simulink model "model_controllers"  (R2019a)
settings: Solver=VariableStepAuto  StartTime=0.0  StopTime=1.2  FixedStep=1e-6  RelTol=1e-5
values from neighbouring files (symbols this model uses):
  Bm = 0.0022    [State_of_Art.m]    (also in results_plotter_one_run20.m)
  Jm = 0.0004    [State_of_Art.m]    (also in results_plotter_one_run20.m)
  k1 = OBL_HSO    [State_of_Art.m]    (also in results_plotter_one_run20.m = kEO)
  k2 = HSO    [State_of_Art.m]    (also in results_plotter_one_run20.m = kPSO)
  k3 = ASO    [State_of_Art.m]    (also in results_plotter_one_run20.m = kSanTLBO)
  k4 = SFS    [State_of_Art.m]    (also in results_plotter_one_run20.m = kDE)
  k5 = GWO    [State_of_Art.m]    (also in results_plotter_one_run20.m = kGA)
  k6 = OBL_HGSO    [results_plotter_one_run20.m]
  k7 = HGSO    [results_plotter_one_run20.m]
  Kb = 0.05    [State_of_Art.m]    (also in results_plotter_one_run20.m)
  Kt = 0.015    [State_of_Art.m]    (also in results_plotter_one_run20.m)
  La = 2.7    [State_of_Art.m]    (also in results_plotter_one_run20.m)
  Ra = 0.4    [State_of_Art.m]    (also in results_plotter_one_run20.m)
libraries: simulink x7, fuzblock x1
settings Model: Creator=Nelson Manuel  LastModifiedBy=Nelson Manuel

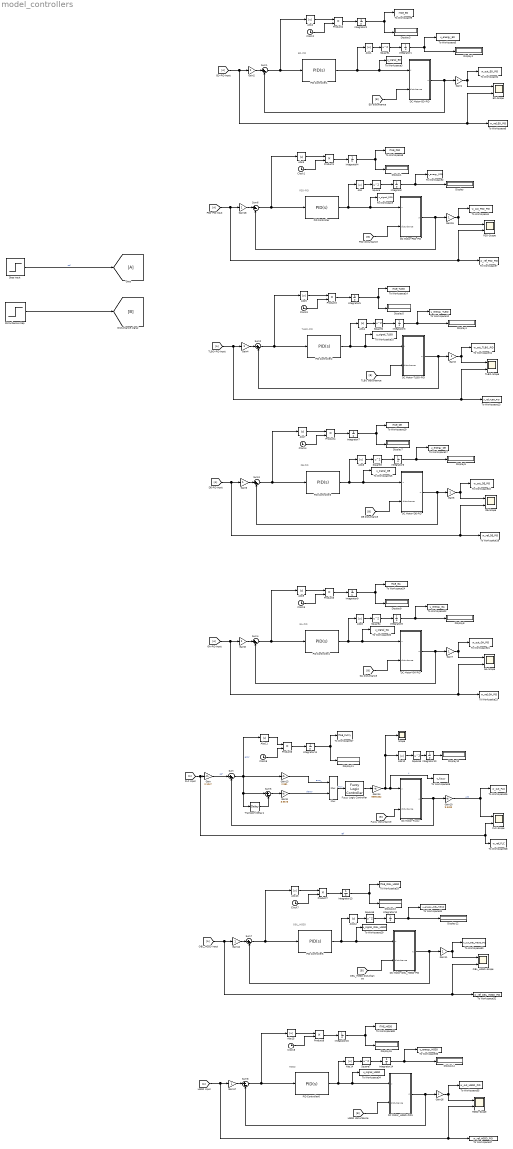
== system model_controllers ==
  note: EO-PID
  note: PSO-PID
  note: TLBO-PID
  note: DE-PID
  note: GA-PID
  note: OBL_HGSO
  note: HGSO
  Abs{,1..15} (16 alike) : Abs
  Clock{1..8} (8 alike) : Clock
  DC Motor-DE-PID : Subsystem
  DC Motor-EO-PID : Subsystem
  DC Motor-Fuzzy : Subsystem
  DC Motor-GA-PID : Subsystem
  DC Motor-OBL_HGSO-PID : Subsystem
  DC Motor-PSO-PID : Subsystem
  DC Motor-TLBO-PID : Subsystem
  DC Motor_HGSO-PID1 : Subsystem
  DE-Scope : Scope  NumInputPorts=2
  Display{,1..15} (16 alike) : Display
  Disturbance step : Step  Time=0  After=0  SampleTime=0
  EO-Scope : Scope  NumInputPorts=2
  FLC-Scope : Scope  NumInputPorts=2
  Fuzzy Logic Controller : fuzblock/Fuzzy Logic  Controller  FIS=FLC_Controller_updated  OutputSampleNumber=101  DataType=double  FuzzifiedInputs=off  RuleFiringStrengths=off  RuleOutputs=off  AggregatedOutputs=off  SimulateUsing=Interpreted execution  OutOfRangeInputValueMessage=none  NoRuleFiredMessage=none  EmptyOutputFuzzySetMessage=none
  GA-Scope : Scope  NumInputPorts=2
  Gain : Gain  Gain=0.1047
  Gain{1..8,11..12,15..18} (14 alike) : Gain
  Gain10 : Gain  Gain=9.5493
  Gain13 : Gain  Gain=2.981
  Gain14 : Gain  Gain=9999.852
  Gain9 : Gain  Gain=8.9578
  HGSO-Scope : Scope  NumInputPorts=2
  Integrator{,1..15} (16 alike) : Integrator
  Mux : Mux  Inputs=2
  OBL_HGSO-Scope : Scope  NumInputPorts=2
  PID Controller : simulink/Continuous/PID Controller  Controller=PID  Form=Parallel  TimeDomain=Continuous-time  SampleTime=-1  IntegratorMethod=Forward Euler  FilterMethod=Forward Euler  ControllerParametersSource=internal  P=k2(1)  I=k2(2)  D=k2(3)  UseFilter=on  N=1000  TunerSelectOption=Transfer Function Based (PID Tuner App)  InitialConditionSource=internal  InitialConditionForIntegrator=0  InitialConditionForFilter=0  DifferentiatorICPrevScaledInput=0  ExternalReset=none  TrackingMode=off  Kt=1  LimitOutput=off  UpperSaturationLimit=inf  LowerSaturationLimit=-inf  LinearizeAsGain=on  AntiWindupMode=none  Kb=1  POutMin=[]  POutMax=[]  IOutMin=[]  IOutMax=[]  DOutMin=[]  DOutMax=[]  NOutMin=[]  NOutMax=[]  SumOutMin=[]  SumOutMax=[]  SaturationOutMin=[]  SaturationOutMax=[]  PParamMin=[]  PParamMax=[]  IParamMin=[]  IParamMax=[]  DParamMin=[]  DParamMax=[]  NParamMin=[]  NParamMax=[]  KbParamMin=[]  KbParamMax=[]  KtParamMin=[]  KtParamMax=[]  KbOutMin=[]  KbOutMax=[]  KtOutMin=[]  KtOutMax=[]  IntegratorOutMin=[]  IntegratorOutMax=[]  FilterOutMin=[]  FilterOutMax=[]  SumI1OutMin=[]  SumI1OutMax=[]  SumI2OutMin=[]  SumI2OutMax=[]  SumI3OutMin=[]  SumI3OutMax=[]  SumI4OutMin=[]  SumI4OutMax=[]  SumDOutMin=[]  SumDOutMax=[]  DifferentiatorOutMin=[]  DifferentiatorOutMax=[]  FilterDiffOutCoefMin=[]  FilterDiffOutCoefMax=[]  ReciprocalOutMin=[]  ReciprocalOutMax=[]  SumDenOutMin=[]  SumDenOutMax=[]  SumNumOutMin=[]  SumNumOutMax=[]  DivideOutMin=[]  DivideOutMax=[]  IntegratorContinuousStateAttributes=''  IntegratorStateMustResolveToSignalObject=off  IntegratorRTWStateStorageClass=Auto  FilterContinuousStateAttributes=''  FilterStateMustResolveToSignalObject=off  FilterRTWStateStorageClass=Auto  ParallelPVariant=InternalParameters  IdealPVariant=Disabled  IVariant=InternalParameters  DVariant=InternalParameters  IntegratorVariant=Continuous  SatVariant=Disabled  AWVariant=Passthrough  PCopyVariant=Disabled  TRVariant=Disabled  FdbkBlocksVariant=Forward  IdealPFdbkVariant=Disabled  SatFdbkVariant=Disabled  DerivativeFilterVariant=ContFilter  NVariant=InternalParameters  NCopyVariant=Disabled  FilterICVariant=InternalICsFilter  IntegratorICVariant=InternalICs  ExternalResetVariant=Disabled  TRSumVariant=Passthrough  SumFdbkVariant=Disabled  SumVariant=Sum_PID
  PID Controller1 : simulink/Continuous/PID Controller  Controller=PID  Form=Parallel  TimeDomain=Continuous-time  SampleTime=-1  IntegratorMethod=Forward Euler  FilterMethod=Forward Euler  ControllerParametersSource=internal  P=k1(1)  I=k1(2)  D=k1(3)  UseFilter=on  N=1000  TunerSelectOption=Transfer Function Based (PID Tuner App)  InitialConditionSource=internal  InitialConditionForIntegrator=0  InitialConditionForFilter=0  DifferentiatorICPrevScaledInput=0  ExternalReset=none  TrackingMode=off  Kt=1  LimitOutput=off  UpperSaturationLimit=inf  LowerSaturationLimit=-inf  LinearizeAsGain=on  AntiWindupMode=none  Kb=1  POutMin=[]  POutMax=[]  IOutMin=[]  IOutMax=[]  DOutMin=[]  DOutMax=[]  NOutMin=[]  NOutMax=[]  SumOutMin=[]  SumOutMax=[]  SaturationOutMin=[]  SaturationOutMax=[]  PParamMin=[]  PParamMax=[]  IParamMin=[]  IParamMax=[]  DParamMin=[]  DParamMax=[]  NParamMin=[]  NParamMax=[]  KbParamMin=[]  KbParamMax=[]  KtParamMin=[]  KtParamMax=[]  KbOutMin=[]  KbOutMax=[]  KtOutMin=[]  KtOutMax=[]  IntegratorOutMin=[]  IntegratorOutMax=[]  FilterOutMin=[]  FilterOutMax=[]  SumI1OutMin=[]  SumI1OutMax=[]  SumI2OutMin=[]  SumI2OutMax=[]  SumI3OutMin=[]  SumI3OutMax=[]  SumI4OutMin=[]  SumI4OutMax=[]  SumDOutMin=[]  SumDOutMax=[]  DifferentiatorOutMin=[]  DifferentiatorOutMax=[]  FilterDiffOutCoefMin=[]  FilterDiffOutCoefMax=[]  ReciprocalOutMin=[]  ReciprocalOutMax=[]  SumDenOutMin=[]  SumDenOutMax=[]  SumNumOutMin=[]  SumNumOutMax=[]  DivideOutMin=[]  DivideOutMax=[]  IntegratorContinuousStateAttributes=''  IntegratorStateMustResolveToSignalObject=off  IntegratorRTWStateStorageClass=Auto  FilterContinuousStateAttributes=''  FilterStateMustResolveToSignalObject=off  FilterRTWStateStorageClass=Auto  ParallelPVariant=InternalParameters  IdealPVariant=Disabled  IVariant=InternalParameters  DVariant=InternalParameters  IntegratorVariant=Continuous  SatVariant=Disabled  AWVariant=Passthrough  PCopyVariant=Disabled  TRVariant=Disabled  FdbkBlocksVariant=Forward  IdealPFdbkVariant=Disabled  SatFdbkVariant=Disabled  DerivativeFilterVariant=ContFilter  NVariant=InternalParameters  NCopyVariant=Disabled  FilterICVariant=InternalICsFilter  IntegratorICVariant=InternalICs  ExternalResetVariant=Disabled  TRSumVariant=Passthrough  SumFdbkVariant=Disabled  SumVariant=Sum_PID
  PID Controller2 : simulink/Continuous/PID Controller  Controller=PID  Form=Parallel  TimeDomain=Continuous-time  SampleTime=-1  IntegratorMethod=Forward Euler  FilterMethod=Forward Euler  ControllerParametersSource=internal  P=k3(1)  I=k3(2)  D=k3(3)  UseFilter=on  N=1000  TunerSelectOption=Transfer Function Based (PID Tuner App)  InitialConditionSource=internal  InitialConditionForIntegrator=0  InitialConditionForFilter=0  DifferentiatorICPrevScaledInput=0  ExternalReset=none  TrackingMode=off  Kt=1  LimitOutput=off  UpperSaturationLimit=inf  LowerSaturationLimit=-inf  LinearizeAsGain=on  AntiWindupMode=none  Kb=1  POutMin=[]  POutMax=[]  IOutMin=[]  IOutMax=[]  DOutMin=[]  DOutMax=[]  NOutMin=[]  NOutMax=[]  SumOutMin=[]  SumOutMax=[]  SaturationOutMin=[]  SaturationOutMax=[]  PParamMin=[]  PParamMax=[]  IParamMin=[]  IParamMax=[]  DParamMin=[]  DParamMax=[]  NParamMin=[]  NParamMax=[]  KbParamMin=[]  KbParamMax=[]  KtParamMin=[]  KtParamMax=[]  KbOutMin=[]  KbOutMax=[]  KtOutMin=[]  KtOutMax=[]  IntegratorOutMin=[]  IntegratorOutMax=[]  FilterOutMin=[]  FilterOutMax=[]  SumI1OutMin=[]  SumI1OutMax=[]  SumI2OutMin=[]  SumI2OutMax=[]  SumI3OutMin=[]  SumI3OutMax=[]  SumI4OutMin=[]  SumI4OutMax=[]  SumDOutMin=[]  SumDOutMax=[]  DifferentiatorOutMin=[]  DifferentiatorOutMax=[]  FilterDiffOutCoefMin=[]  FilterDiffOutCoefMax=[]  ReciprocalOutMin=[]  ReciprocalOutMax=[]  SumDenOutMin=[]  SumDenOutMax=[]  SumNumOutMin=[]  SumNumOutMax=[]  DivideOutMin=[]  DivideOutMax=[]  IntegratorContinuousStateAttributes=''  IntegratorStateMustResolveToSignalObject=off  IntegratorRTWStateStorageClass=Auto  FilterContinuousStateAttributes=''  FilterStateMustResolveToSignalObject=off  FilterRTWStateStorageClass=Auto  ParallelPVariant=InternalParameters  IdealPVariant=Disabled  IVariant=InternalParameters  DVariant=InternalParameters  IntegratorVariant=Continuous  SatVariant=Disabled  AWVariant=Passthrough  PCopyVariant=Disabled  TRVariant=Disabled  FdbkBlocksVariant=Forward  IdealPFdbkVariant=Disabled  SatFdbkVariant=Disabled  DerivativeFilterVariant=ContFilter  NVariant=InternalParameters  NCopyVariant=Disabled  FilterICVariant=InternalICsFilter  IntegratorICVariant=InternalICs  ExternalResetVariant=Disabled  TRSumVariant=Passthrough  SumFdbkVariant=Disabled  SumVariant=Sum_PID
  PID Controller3 : simulink/Continuous/PID Controller  Controller=PID  Form=Parallel  TimeDomain=Continuous-time  SampleTime=-1  IntegratorMethod=Forward Euler  FilterMethod=Forward Euler  ControllerParametersSource=internal  P=k4(1)  I=k4(2)  D=k4(3)  UseFilter=on  N=1000  TunerSelectOption=Transfer Function Based (PID Tuner App)  InitialConditionSource=internal  InitialConditionForIntegrator=0  InitialConditionForFilter=0  DifferentiatorICPrevScaledInput=0  ExternalReset=none  TrackingMode=off  Kt=1  LimitOutput=off  UpperSaturationLimit=inf  LowerSaturationLimit=-inf  LinearizeAsGain=on  AntiWindupMode=none  Kb=1  POutMin=[]  POutMax=[]  IOutMin=[]  IOutMax=[]  DOutMin=[]  DOutMax=[]  NOutMin=[]  NOutMax=[]  SumOutMin=[]  SumOutMax=[]  SaturationOutMin=[]  SaturationOutMax=[]  PParamMin=[]  PParamMax=[]  IParamMin=[]  IParamMax=[]  DParamMin=[]  DParamMax=[]  NParamMin=[]  NParamMax=[]  KbParamMin=[]  KbParamMax=[]  KtParamMin=[]  KtParamMax=[]  KbOutMin=[]  KbOutMax=[]  KtOutMin=[]  KtOutMax=[]  IntegratorOutMin=[]  IntegratorOutMax=[]  FilterOutMin=[]  FilterOutMax=[]  SumI1OutMin=[]  SumI1OutMax=[]  SumI2OutMin=[]  SumI2OutMax=[]  SumI3OutMin=[]  SumI3OutMax=[]  SumI4OutMin=[]  SumI4OutMax=[]  SumDOutMin=[]  SumDOutMax=[]  DifferentiatorOutMin=[]  DifferentiatorOutMax=[]  FilterDiffOutCoefMin=[]  FilterDiffOutCoefMax=[]  ReciprocalOutMin=[]  ReciprocalOutMax=[]  SumDenOutMin=[]  SumDenOutMax=[]  SumNumOutMin=[]  SumNumOutMax=[]  DivideOutMin=[]  DivideOutMax=[]  IntegratorContinuousStateAttributes=''  IntegratorStateMustResolveToSignalObject=off  IntegratorRTWStateStorageClass=Auto  FilterContinuousStateAttributes=''  FilterStateMustResolveToSignalObject=off  FilterRTWStateStorageClass=Auto  ParallelPVariant=InternalParameters  IdealPVariant=Disabled  IVariant=InternalParameters  DVariant=InternalParameters  IntegratorVariant=Continuous  SatVariant=Disabled  AWVariant=Passthrough  PCopyVariant=Disabled  TRVariant=Disabled  FdbkBlocksVariant=Forward  IdealPFdbkVariant=Disabled  SatFdbkVariant=Disabled  DerivativeFilterVariant=ContFilter  NVariant=InternalParameters  NCopyVariant=Disabled  FilterICVariant=InternalICsFilter  IntegratorICVariant=InternalICs  ExternalResetVariant=Disabled  TRSumVariant=Passthrough  SumFdbkVariant=Disabled  SumVariant=Sum_PID
  PID Controller4 : simulink/Continuous/PID Controller  Controller=PID  Form=Parallel  TimeDomain=Continuous-time  SampleTime=-1  IntegratorMethod=Forward Euler  FilterMethod=Forward Euler  ControllerParametersSource=internal  P=k5(1)  I=k5(2)  D=k5(3)  UseFilter=on  N=1000  TunerSelectOption=Transfer Function Based (PID Tuner App)  InitialConditionSource=internal  InitialConditionForIntegrator=0  InitialConditionForFilter=0  DifferentiatorICPrevScaledInput=0  ExternalReset=none  TrackingMode=off  Kt=1  LimitOutput=off  UpperSaturationLimit=inf  LowerSaturationLimit=-inf  LinearizeAsGain=on  AntiWindupMode=none  Kb=1  POutMin=[]  POutMax=[]  IOutMin=[]  IOutMax=[]  DOutMin=[]  DOutMax=[]  NOutMin=[]  NOutMax=[]  SumOutMin=[]  SumOutMax=[]  SaturationOutMin=[]  SaturationOutMax=[]  PParamMin=[]  PParamMax=[]  IParamMin=[]  IParamMax=[]  DParamMin=[]  DParamMax=[]  NParamMin=[]  NParamMax=[]  KbParamMin=[]  KbParamMax=[]  KtParamMin=[]  KtParamMax=[]  KbOutMin=[]  KbOutMax=[]  KtOutMin=[]  KtOutMax=[]  IntegratorOutMin=[]  IntegratorOutMax=[]  FilterOutMin=[]  FilterOutMax=[]  SumI1OutMin=[]  SumI1OutMax=[]  SumI2OutMin=[]  SumI2OutMax=[]  SumI3OutMin=[]  SumI3OutMax=[]  SumI4OutMin=[]  SumI4OutMax=[]  SumDOutMin=[]  SumDOutMax=[]  DifferentiatorOutMin=[]  DifferentiatorOutMax=[]  FilterDiffOutCoefMin=[]  FilterDiffOutCoefMax=[]  ReciprocalOutMin=[]  ReciprocalOutMax=[]  SumDenOutMin=[]  SumDenOutMax=[]  SumNumOutMin=[]  SumNumOutMax=[]  DivideOutMin=[]  DivideOutMax=[]  IntegratorContinuousStateAttributes=''  IntegratorStateMustResolveToSignalObject=off  IntegratorRTWStateStorageClass=Auto  FilterContinuousStateAttributes=''  FilterStateMustResolveToSignalObject=off  FilterRTWStateStorageClass=Auto  ParallelPVariant=InternalParameters  IdealPVariant=Disabled  IVariant=InternalParameters  DVariant=InternalParameters  IntegratorVariant=Continuous  SatVariant=Disabled  AWVariant=Passthrough  PCopyVariant=Disabled  TRVariant=Disabled  FdbkBlocksVariant=Forward  IdealPFdbkVariant=Disabled  SatFdbkVariant=Disabled  DerivativeFilterVariant=ContFilter  NVariant=InternalParameters  NCopyVariant=Disabled  FilterICVariant=InternalICsFilter  IntegratorICVariant=InternalICs  ExternalResetVariant=Disabled  TRSumVariant=Passthrough  SumFdbkVariant=Disabled  SumVariant=Sum_PID
  PID Controller5 : simulink/Continuous/PID Controller  Controller=PID  Form=Parallel  TimeDomain=Continuous-time  SampleTime=-1  IntegratorMethod=Forward Euler  FilterMethod=Forward Euler  ControllerParametersSource=internal  P=k6(1)  I=k6(2)  D=k6(3)  UseFilter=on  N=1000  TunerSelectOption=Transfer Function Based (PID Tuner App)  InitialConditionSource=internal  InitialConditionForIntegrator=0  InitialConditionForFilter=0  DifferentiatorICPrevScaledInput=0  ExternalReset=none  TrackingMode=off  Kt=1  LimitOutput=off  UpperSaturationLimit=inf  LowerSaturationLimit=-inf  LinearizeAsGain=on  AntiWindupMode=none  Kb=1  POutMin=[]  POutMax=[]  IOutMin=[]  IOutMax=[]  DOutMin=[]  DOutMax=[]  NOutMin=[]  NOutMax=[]  SumOutMin=[]  SumOutMax=[]  SaturationOutMin=[]  SaturationOutMax=[]  PParamMin=[]  PParamMax=[]  IParamMin=[]  IParamMax=[]  DParamMin=[]  DParamMax=[]  NParamMin=[]  NParamMax=[]  KbParamMin=[]  KbParamMax=[]  KtParamMin=[]  KtParamMax=[]  KbOutMin=[]  KbOutMax=[]  KtOutMin=[]  KtOutMax=[]  IntegratorOutMin=[]  IntegratorOutMax=[]  FilterOutMin=[]  FilterOutMax=[]  SumI1OutMin=[]  SumI1OutMax=[]  SumI2OutMin=[]  SumI2OutMax=[]  SumI3OutMin=[]  SumI3OutMax=[]  SumI4OutMin=[]  SumI4OutMax=[]  SumDOutMin=[]  SumDOutMax=[]  DifferentiatorOutMin=[]  DifferentiatorOutMax=[]  FilterDiffOutCoefMin=[]  FilterDiffOutCoefMax=[]  ReciprocalOutMin=[]  ReciprocalOutMax=[]  SumDenOutMin=[]  SumDenOutMax=[]  SumNumOutMin=[]  SumNumOutMax=[]  DivideOutMin=[]  DivideOutMax=[]  IntegratorContinuousStateAttributes=''  IntegratorStateMustResolveToSignalObject=off  IntegratorRTWStateStorageClass=Auto  FilterContinuousStateAttributes=''  FilterStateMustResolveToSignalObject=off  FilterRTWStateStorageClass=Auto  ParallelPVariant=InternalParameters  IdealPVariant=Disabled  IVariant=InternalParameters  DVariant=InternalParameters  IntegratorVariant=Continuous  SatVariant=Disabled  AWVariant=Passthrough  PCopyVariant=Disabled  TRVariant=Disabled  FdbkBlocksVariant=Forward  IdealPFdbkVariant=Disabled  SatFdbkVariant=Disabled  DerivativeFilterVariant=ContFilter  NVariant=InternalParameters  NCopyVariant=Disabled  FilterICVariant=InternalICsFilter  IntegratorICVariant=InternalICs  ExternalResetVariant=Disabled  TRSumVariant=Passthrough  SumFdbkVariant=Disabled  SumVariant=Sum_PID
  PID Controller6 : simulink/Continuous/PID Controller  Controller=PID  Form=Parallel  TimeDomain=Continuous-time  SampleTime=-1  IntegratorMethod=Forward Euler  FilterMethod=Forward Euler  ControllerParametersSource=internal  P=k7(1)  I=k7(2)  D=k7(3)  UseFilter=on  N=1000  TunerSelectOption=Transfer Function Based (PID Tuner App)  InitialConditionSource=internal  InitialConditionForIntegrator=0  InitialConditionForFilter=0  DifferentiatorICPrevScaledInput=0  ExternalReset=none  TrackingMode=off  Kt=1  LimitOutput=off  UpperSaturationLimit=inf  LowerSaturationLimit=-inf  LinearizeAsGain=on  AntiWindupMode=none  Kb=1  POutMin=[]  POutMax=[]  IOutMin=[]  IOutMax=[]  DOutMin=[]  DOutMax=[]  NOutMin=[]  NOutMax=[]  SumOutMin=[]  SumOutMax=[]  SaturationOutMin=[]  SaturationOutMax=[]  PParamMin=[]  PParamMax=[]  IParamMin=[]  IParamMax=[]  DParamMin=[]  DParamMax=[]  NParamMin=[]  NParamMax=[]  KbParamMin=[]  KbParamMax=[]  KtParamMin=[]  KtParamMax=[]  KbOutMin=[]  KbOutMax=[]  KtOutMin=[]  KtOutMax=[]  IntegratorOutMin=[]  IntegratorOutMax=[]  FilterOutMin=[]  FilterOutMax=[]  SumI1OutMin=[]  SumI1OutMax=[]  SumI2OutMin=[]  SumI2OutMax=[]  SumI3OutMin=[]  SumI3OutMax=[]  SumI4OutMin=[]  SumI4OutMax=[]  SumDOutMin=[]  SumDOutMax=[]  DifferentiatorOutMin=[]  DifferentiatorOutMax=[]  FilterDiffOutCoefMin=[]  FilterDiffOutCoefMax=[]  ReciprocalOutMin=[]  ReciprocalOutMax=[]  SumDenOutMin=[]  SumDenOutMax=[]  SumNumOutMin=[]  SumNumOutMax=[]  DivideOutMin=[]  DivideOutMax=[]  IntegratorContinuousStateAttributes=''  IntegratorStateMustResolveToSignalObject=off  IntegratorRTWStateStorageClass=Auto  FilterContinuousStateAttributes=''  FilterStateMustResolveToSignalObject=off  FilterRTWStateStorageClass=Auto  ParallelPVariant=InternalParameters  IdealPVariant=Disabled  IVariant=InternalParameters  DVariant=InternalParameters  IntegratorVariant=Continuous  SatVariant=Disabled  AWVariant=Passthrough  PCopyVariant=Disabled  TRVariant=Disabled  FdbkBlocksVariant=Forward  IdealPFdbkVariant=Disabled  SatFdbkVariant=Disabled  DerivativeFilterVariant=ContFilter  NVariant=InternalParameters  NCopyVariant=Disabled  FilterICVariant=InternalICsFilter  IntegratorICVariant=InternalICs  ExternalResetVariant=Disabled  TRSumVariant=Passthrough  SumFdbkVariant=Disabled  SumVariant=Sum_PID
  PSO-Scope : Scope  NumInputPorts=2
  Product{1..8} (8 alike) : Product
  Scope : Scope
  Square{,1..7} (8 alike) : Math  Operator=square  SaturateOnIntegerOverflow=on
  Step Input : Step  Time=0  SampleTime=0
  Sum{,1..8} (9 alike) : Sum  Inputs=|+-
  TLBO-Scope : Scope  NumInputPorts=2
  To Workspace : ToWorkspace  VariableName=u_signal_PSO  SaveFormat=Timeseries  SampleTime=-1
  To Workspace1 : ToWorkspace  VariableName=w_out_PSO_PID  SaveFormat=Timeseries  SampleTime=-1
  To Workspace10 : ToWorkspace  VariableName=u_signal_TLBO  SaveFormat=Timeseries  SampleTime=-1
  To Workspace11 : ToWorkspace  VariableName=w_out_TLBO_PID  SaveFormat=Timeseries  SampleTime=-1
  To Workspace12 : ToWorkspace  VariableName=u_energy_TLBO  SaveFormat=Timeseries  SampleTime=-1
  To Workspace13 : ToWorkspace  VariableName=w_ref_TLBO_PID  SaveFormat=Timeseries  SampleTime=-1
  To Workspace14 : ToWorkspace  VariableName=ITAE_TLBO  SaveFormat=Timeseries  SampleTime=-1
  To Workspace15 : ToWorkspace  VariableName=u_signal_DE  SaveFormat=Timeseries  SampleTime=-1
  To Workspace16 : ToWorkspace  VariableName=w_out_DE_PID  SaveFormat=Timeseries  SampleTime=-1
  To Workspace17 : ToWorkspace  VariableName=u_energy_DE  SaveFormat=Timeseries  SampleTime=-1
  To Workspace18 : ToWorkspace  VariableName=w_ref_DE_PID  SaveFormat=Timeseries  SampleTime=-1
  To Workspace19 : ToWorkspace  VariableName=ITAE_DE  SaveFormat=Timeseries  SampleTime=-1
  To Workspace2 : ToWorkspace  VariableName=u_energy_PSO  SaveFormat=Timeseries  SampleTime=-1
  To Workspace20 : ToWorkspace  VariableName=u_signal_GA  SaveFormat=Timeseries  SampleTime=-1
  To Workspace21 : ToWorkspace  VariableName=w_out_GA_PID  SaveFormat=Timeseries  SampleTime=-1
  To Workspace22 : ToWorkspace  VariableName=u_energy_GA  SaveFormat=Timeseries  SampleTime=-1
  To Workspace23 : ToWorkspace  VariableName=w_ref_GA_PID  SaveFormat=Timeseries  SampleTime=-1
  To Workspace24 : ToWorkspace  VariableName=ITAE_GA  SaveFormat=Timeseries  SampleTime=-1
  To Workspace25 : ToWorkspace  VariableName=w_out_FLC  SaveFormat=Timeseries  SampleTime=-1
  To Workspace26 : ToWorkspace  VariableName=u_fuzzy  SaveFormat=Timeseries  SampleTime=-1
  To Workspace27 : ToWorkspace  VariableName=ITAE_Fuzzy  SaveFormat=Timeseries  SampleTime=-1
  To Workspace28 : ToWorkspace  VariableName=w_ref_FLC  SaveFormat=Timeseries  SampleTime=-1
  To Workspace29 : ToWorkspace  VariableName=u_signal_OBL_HGSO  SaveFormat=Timeseries  SampleTime=-1
  To Workspace3 : ToWorkspace  VariableName=u_signal_EO  SaveFormat=Timeseries  SampleTime=-1
  To Workspace30 : ToWorkspace  VariableName=w_out_OBL_HGSO_PID  SaveFormat=Timeseries  SampleTime=-1
  To Workspace31 : ToWorkspace  VariableName=u_energy_OBL_HGSO  SaveFormat=Timeseries  SampleTime=-1
  To Workspace32 : ToWorkspace  VariableName=w_ref_OBL_HGSO_PID  SaveFormat=Timeseries  SampleTime=-1
  To Workspace33 : ToWorkspace  VariableName=ITAE_OBL_HGSO  SaveFormat=Timeseries  SampleTime=-1
  To Workspace34 : ToWorkspace  VariableName=u_signal_HGSO  SaveFormat=Timeseries  SampleTime=-1
  To Workspace35 : ToWorkspace  VariableName=w_out_HGSO_PID  SaveFormat=Timeseries  SampleTime=-1
  To Workspace36 : ToWorkspace  VariableName=u_energy_HGSO  SaveFormat=Timeseries  SampleTime=-1
  To Workspace37 : ToWorkspace  VariableName=w_ref_HGSO_PID  SaveFormat=Timeseries  SampleTime=-1
  To Workspace38 : ToWorkspace  VariableName=ITAE_HGSO  SaveFormat=Timeseries  SampleTime=-1
  To Workspace4 : ToWorkspace  VariableName=w_out_EO_PID  SaveFormat=Timeseries  SampleTime=-1
  To Workspace5 : ToWorkspace  VariableName=u_energy_EO  SaveFormat=Timeseries  SampleTime=-1
  To Workspace6 : ToWorkspace  VariableName=w_ref_EO_PID  SaveFormat=Timeseries  SampleTime=-1
  To Workspace7 : ToWorkspace  VariableName=w_ref_PSO_PID  SaveFormat=Timeseries  SampleTime=-1
  To Workspace8 : ToWorkspace  VariableName=ITAE_PSO  SaveFormat=Timeseries  SampleTime=-1
  To Workspace9 : ToWorkspace  VariableName=ITAE_EO  SaveFormat=Timeseries  SampleTime=-1
  Transport Delay1 : TransportDelay  DelayTime=0.00056797432  BufferSize=2048
  wires:
  [A] -> Gain18/1, To Workspace7/1, PSO-Scope/2
  [B] -> DC Motor-PSO-PID/2(disturbance)
  Clock1/1 -> Product1/2
  Gain18/1 -> Sum6/1
  Gain15/1 -> PSO-Scope/1, To Workspace1/1
  Product1/1 -> Integrator4/1
  Integrator4/1 -> To Workspace8/1, Display1/1
  Abs3/1 -> Product1/1
  Sum6/1 -> PID Controller/1, Abs3/1
  DC Motor-PSO-PID/1(w) -> Gain15/1, Sum6/2
  Disturbance step/1 -> [B]
  Step Input/1 -> [A]  "ref"
  Integrator/1 -> To Workspace2/1, Display/1
  PID Controller/1 -> Abs/1, To Workspace/1, DC Motor-PSO-PID/1(u)
  Square/1 -> Integrator/1
  Abs/1 -> Square/1
  Square1/1 -> Integrator1/1
  Sum1/1 -> PID Controller1/1, Abs2/1
  DC Motor-EO-PID/1(w) -> Gain1/1, Sum1/2
  PID Controller1/1 -> Abs1/1, To Workspace3/1, DC Motor-EO-PID/1(u)
  Gain1/1 -> EO-Scope/1, To Workspace4/1
  Integrator2/1 -> To Workspace9/1, Display3/1
  Product2/1 -> Integrator2/1
  Abs2/1 -> Product2/1
  Clock2/1 -> Product2/2
  Gain2/1 -> Sum1/1
  Integrator1/1 -> To Workspace5/1, Display2/1
  [B] -> DC Motor-EO-PID/2(disturbance)
  [A] -> Gain2/1, To Workspace6/1, EO-Scope/2
  Abs1/1 -> Square1/1
  Square2/1 -> Integrator3/1
  Sum2/1 -> PID Controller2/1, Abs5/1
  DC Motor-TLBO-PID/1(w) -> Gain3/1, Sum2/2
  PID Controller2/1 -> Abs4/1, To Workspace10/1, DC Motor-TLBO-PID/1(u)
  Gain3/1 -> TLBO-Scope/1, To Workspace11/1
  Integrator5/1 -> To Workspace14/1, Display5/1
  Product3/1 -> Integrator5/1
  Abs5/1 -> Product3/1
  Clock3/1 -> Product3/2
  Gain4/1 -> Sum2/1
  Integrator3/1 -> To Workspace12/1, Display4/1
  [B] -> DC Motor-TLBO-PID/2(disturbance)
  [A] -> Gain4/1, To Workspace13/1, TLBO-Scope/2
  Abs4/1 -> Square2/1
  [A] -> Gain6/1, To Workspace18/1, DE-Scope/2
  Abs6/1 -> Square3/1
  [B] -> DC Motor-DE-PID/2(disturbance)
  Integrator6/1 -> To Workspace17/1, Display6/1
  Product4/1 -> Integrator7/1
  Abs7/1 -> Product4/1
  Gain6/1 -> Sum3/1
  Integrator7/1 -> To Workspace19/1, Display7/1
  Gain5/1 -> DE-Scope/1, To Workspace16/1
  DC Motor-DE-PID/1(w) -> Gain5/1, Sum3/2
  Clock4/1 -> Product4/2
  Sum3/1 -> PID Controller3/1, Abs7/1
  Square3/1 -> Integrator6/1
  DC Motor-GA-PID/1(w) -> Gain7/1, Sum4/2
  Square4/1 -> Integrator8/1
  Sum4/1 -> PID Controller4/1, Abs9/1
  Clock5/1 -> Product5/2
  PID Controller4/1 -> Abs8/1, To Workspace20/1, DC Motor-GA-PID/1(u)
  Gain7/1 -> GA-Scope/1, To Workspace21/1
  Integrator9/1 -> To Workspace24/1, Display9/1
  Product5/1 -> Integrator9/1
  Gain8/1 -> Sum4/1
  Integrator8/1 -> To Workspace22/1, Display8/1
  Abs9/1 -> Product5/1
  [B] -> DC Motor-GA-PID/2(disturbance)
  [A] -> Gain8/1, To Workspace23/1, GA-Scope/2
  Abs8/1 -> Square4/1
  Integrator10/1 -> Display10/1
  Sum5/1 -> Gain9/1
  Gain14/1 -> Scope/1, Abs10/1, To Workspace26/1, DC Motor-Fuzzy/1(u)  "u"
  Abs10/1 -> Square5/1
  Fuzzy Logic Controller/1 -> Gain14/1
  [B] -> DC Motor-Fuzzy/2(disturbance)
  DC Motor-Fuzzy/1(w) -> Gain10/1, Sum/2
  Square5/1 -> Integrator10/1
  Gain9/1 -> Mux/2  "derror"
  [A] -> FLC-Scope/2, To Workspace28/1, Gain/1  "ref"
  Integrator11/1 -> To Workspace27/1, Display11/1
  Clock6/1 -> Product6/2
  Gain/1 -> Sum/1  "ref"
  Transport Delay1/1 -> Sum5/2
  Mux/1 -> Fuzzy Logic Controller/1  "mux"
  Gain13/1 -> Mux/1  "error_"
  Product6/1 -> Integrator11/1
  Abs11/1 -> Product6/1
  Gain10/1 -> FLC-Scope/1, To Workspace25/1  "w(t)"
  Sum/1 -> Transport Delay1/1, Sum5/1, Gain13/1, Abs11/1  "error"
  PID Controller3/1 -> Abs6/1, To Workspace15/1, DC Motor-DE-PID/1(u)
  PID Controller5/1 -> Abs12/1, To Workspace29/1, DC Motor-OBL_HGSO-PID/1(u)
  Product7/1 -> Integrator13/1
  Gain12/1 -> Sum7/1
  [A] -> Gain12/1, OBL_HGSO-Scope/2, To Workspace32/1
  DC Motor-OBL_HGSO-PID/1(w) -> Gain11/1, Sum7/2
  [B] -> DC Motor-OBL_HGSO-PID/2(disturbance)
  Abs12/1 -> Square6/1
  Gain11/1 -> OBL_HGSO-Scope/1, To Workspace30/1
  Integrator13/1 -> To Workspace33/1, Display13/1
  Abs13/1 -> Product7/1
  Integrator12/1 -> To Workspace31/1, Display12/1
  Square6/1 -> Integrator12/1
  Sum7/1 -> PID Controller5/1, Abs13/1
  Clock7/1 -> Product7/2
  Clock8/1 -> Product8/2
  Abs15/1 -> Product8/1
  Integrator15/1 -> To Workspace38/1, Display15/1
  Integrator14/1 -> To Workspace36/1, Display14/1
  Sum8/1 -> PID Controller6/1, Abs15/1
  Gain16/1 -> HGSO-Scope/1, To Workspace35/1
  DC Motor_HGSO-PID1/1(w) -> Gain16/1, Sum8/2
  [B] -> DC Motor_HGSO-PID1/2(disturbance)
  [A] -> Gain17/1, HGSO-Scope/2, To Workspace37/1
  Square7/1 -> Integrator14/1
  Product8/1 -> Integrator15/1
  PID Controller6/1 -> Abs14/1, To Workspace34/1, DC Motor_HGSO-PID1/1(u)
  Abs14/1 -> Square7/1
  Gain17/1 -> Sum8/1

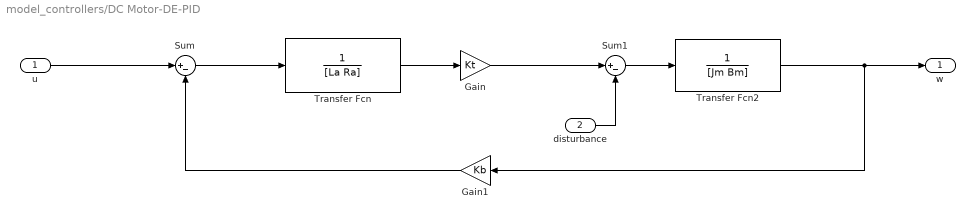
== system model_controllers/DC Motor-DE-PID ==
  u : Inport
  disturbance : Inport  Port=2
  Gain : Gain  Gain=Kt
  Gain1 : Gain  Gain=Kb
  Sum : Sum  Inputs=|+-
  Sum1 : Sum  Inputs=|+-
  Transfer Fcn : TransferFcn  Denominator=[La Ra]
  Transfer Fcn2 : TransferFcn  Denominator=[Jm Bm]
  w : Outport
  wires:
  Sum/1 -> Transfer Fcn/1
  Transfer Fcn/1 -> Gain/1
  Gain/1 -> Sum1/1
  Sum1/1 -> Transfer Fcn2/1
  Gain1/1 -> Sum/2
  Transfer Fcn2/1 -> w/1, Gain1/1
  disturbance/1 -> Sum1/2
  u/1 -> Sum/1

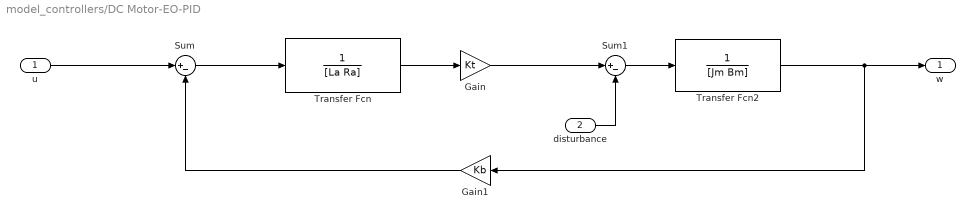
== system model_controllers/DC Motor-EO-PID ==
  u : Inport
  disturbance : Inport  Port=2
  Gain : Gain  Gain=Kt
  Gain1 : Gain  Gain=Kb
  Sum : Sum  Inputs=|+-
  Sum1 : Sum  Inputs=|+-
  Transfer Fcn : TransferFcn  Denominator=[La Ra]
  Transfer Fcn2 : TransferFcn  Denominator=[Jm Bm]
  w : Outport
  wires:
  Sum/1 -> Transfer Fcn/1
  Transfer Fcn/1 -> Gain/1
  Gain/1 -> Sum1/1
  Sum1/1 -> Transfer Fcn2/1
  Gain1/1 -> Sum/2
  Transfer Fcn2/1 -> w/1, Gain1/1
  disturbance/1 -> Sum1/2
  u/1 -> Sum/1

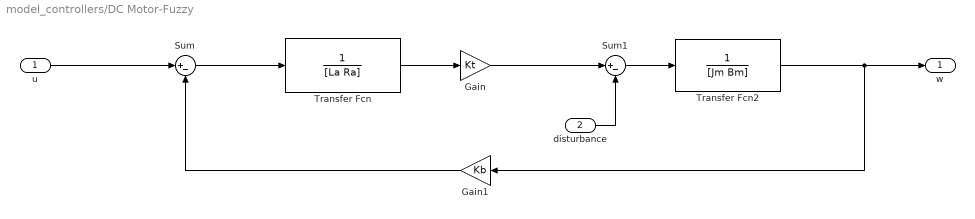
== system model_controllers/DC Motor-Fuzzy ==
  u : Inport
  disturbance : Inport  Port=2
  Gain : Gain  Gain=Kt
  Gain1 : Gain  Gain=Kb
  Sum : Sum  Inputs=|+-
  Sum1 : Sum  Inputs=|+-
  Transfer Fcn : TransferFcn  Denominator=[La Ra]
  Transfer Fcn2 : TransferFcn  Denominator=[Jm Bm]
  w : Outport
  wires:
  Sum/1 -> Transfer Fcn/1
  Transfer Fcn2/1 -> w/1, Gain1/1
  disturbance/1 -> Sum1/2
  Gain/1 -> Sum1/1
  Gain1/1 -> Sum/2
  u/1 -> Sum/1
  Transfer Fcn/1 -> Gain/1
  Sum1/1 -> Transfer Fcn2/1

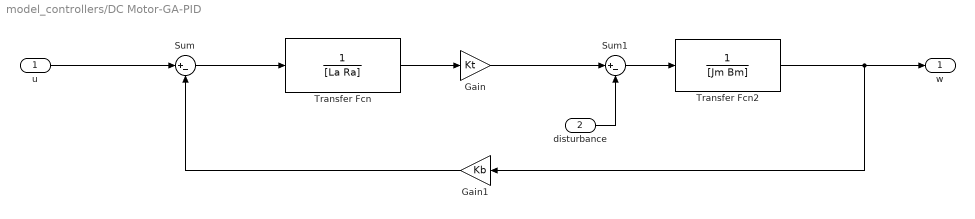
== system model_controllers/DC Motor-GA-PID ==
  u : Inport
  disturbance : Inport  Port=2
  Gain : Gain  Gain=Kt
  Gain1 : Gain  Gain=Kb
  Sum : Sum  Inputs=|+-
  Sum1 : Sum  Inputs=|+-
  Transfer Fcn : TransferFcn  Denominator=[La Ra]
  Transfer Fcn2 : TransferFcn  Denominator=[Jm Bm]
  w : Outport
  wires:
  Sum/1 -> Transfer Fcn/1
  Transfer Fcn/1 -> Gain/1
  Gain/1 -> Sum1/1
  Sum1/1 -> Transfer Fcn2/1
  Gain1/1 -> Sum/2
  Transfer Fcn2/1 -> w/1, Gain1/1
  disturbance/1 -> Sum1/2
  u/1 -> Sum/1

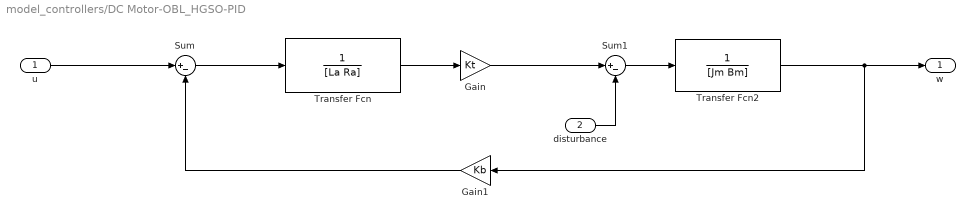
== system model_controllers/DC Motor-OBL_HGSO-PID ==
  u : Inport
  disturbance : Inport  Port=2
  Gain : Gain  Gain=Kt
  Gain1 : Gain  Gain=Kb
  Sum : Sum  Inputs=|+-
  Sum1 : Sum  Inputs=|+-
  Transfer Fcn : TransferFcn  Denominator=[La Ra]
  Transfer Fcn2 : TransferFcn  Denominator=[Jm Bm]
  w : Outport
  wires:
  Sum/1 -> Transfer Fcn/1
  Transfer Fcn/1 -> Gain/1
  Gain/1 -> Sum1/1
  Sum1/1 -> Transfer Fcn2/1
  Gain1/1 -> Sum/2
  Transfer Fcn2/1 -> w/1, Gain1/1
  disturbance/1 -> Sum1/2
  u/1 -> Sum/1

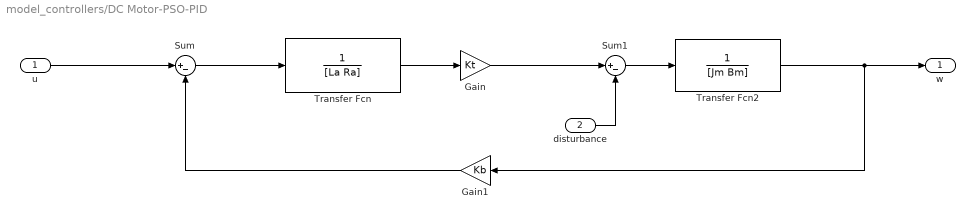
== system model_controllers/DC Motor-PSO-PID ==
  u : Inport
  disturbance : Inport  Port=2
  Gain : Gain  Gain=Kt
  Gain1 : Gain  Gain=Kb
  Sum : Sum  Inputs=|+-
  Sum1 : Sum  Inputs=|+-
  Transfer Fcn : TransferFcn  Denominator=[La Ra]
  Transfer Fcn2 : TransferFcn  Denominator=[Jm Bm]
  w : Outport
  wires:
  Sum/1 -> Transfer Fcn/1
  Transfer Fcn/1 -> Gain/1
  Gain/1 -> Sum1/1
  Sum1/1 -> Transfer Fcn2/1
  Gain1/1 -> Sum/2
  Transfer Fcn2/1 -> w/1, Gain1/1
  disturbance/1 -> Sum1/2
  u/1 -> Sum/1

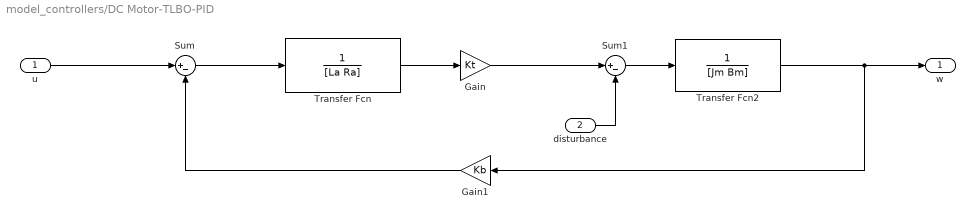
== system model_controllers/DC Motor-TLBO-PID ==
  u : Inport
  disturbance : Inport  Port=2
  Gain : Gain  Gain=Kt
  Gain1 : Gain  Gain=Kb
  Sum : Sum  Inputs=|+-
  Sum1 : Sum  Inputs=|+-
  Transfer Fcn : TransferFcn  Denominator=[La Ra]
  Transfer Fcn2 : TransferFcn  Denominator=[Jm Bm]
  w : Outport
  wires:
  Sum/1 -> Transfer Fcn/1
  Transfer Fcn/1 -> Gain/1
  Gain/1 -> Sum1/1
  Sum1/1 -> Transfer Fcn2/1
  Gain1/1 -> Sum/2
  Transfer Fcn2/1 -> w/1, Gain1/1
  disturbance/1 -> Sum1/2
  u/1 -> Sum/1

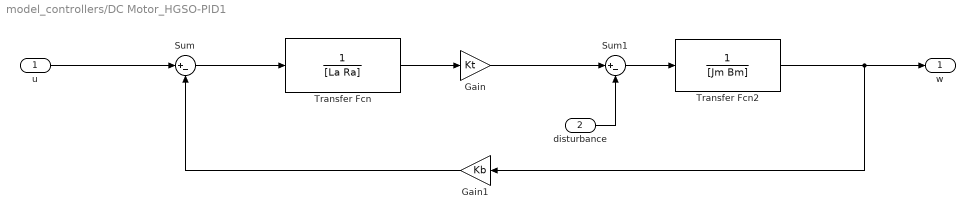
== system model_controllers/DC Motor_HGSO-PID1 ==
  u : Inport
  disturbance : Inport  Port=2
  Gain : Gain  Gain=Kt
  Gain1 : Gain  Gain=Kb
  Sum : Sum  Inputs=|+-
  Sum1 : Sum  Inputs=|+-
  Transfer Fcn : TransferFcn  Denominator=[La Ra]
  Transfer Fcn2 : TransferFcn  Denominator=[Jm Bm]
  w : Outport
  wires:
  Sum/1 -> Transfer Fcn/1
  Transfer Fcn/1 -> Gain/1
  Gain/1 -> Sum1/1
  Sum1/1 -> Transfer Fcn2/1
  Gain1/1 -> Sum/2
  Transfer Fcn2/1 -> w/1, Gain1/1
  disturbance/1 -> Sum1/2
  u/1 -> Sum/1
